simulink model "Bioloid_FK"  (R2013a)
settings: Solver=ode45  StartTime=0.0  StopTime=inf  RelTol=1e-3
undefined symbols (not defined in the file or in its folder): ToSimulink_Bioloid_FK_ST, ToSimulink_Bioloid_Signals2VRML
libraries: simulink x24, vrlib x1
settings Model: Creator=Jose Angel Rangel  LastModifiedBy=Angel

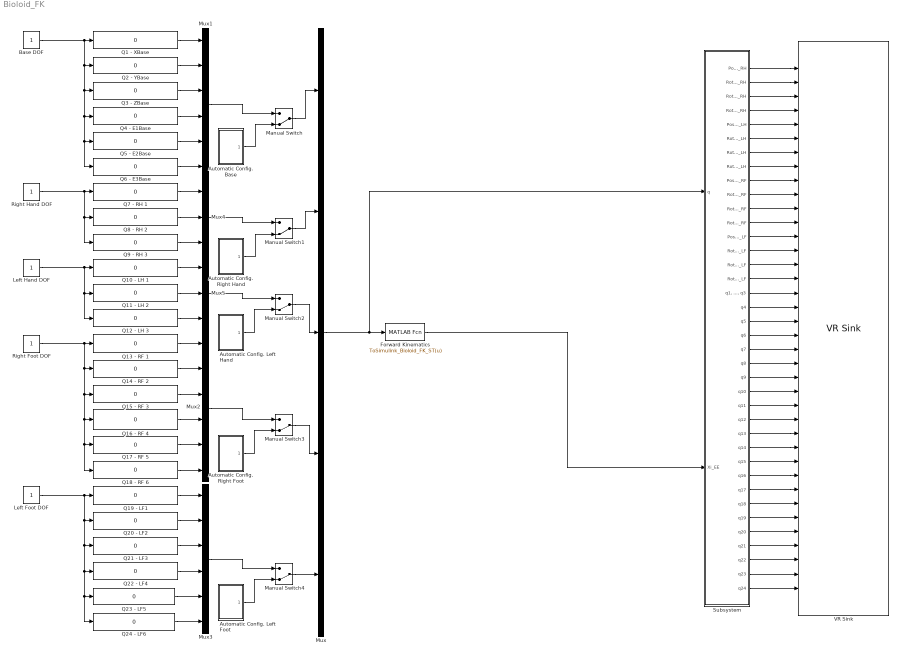
== system Bioloid_FK ==
  Automatic Config. Base : Subsystem
  Automatic Config. Left Foot : Subsystem
  Automatic Config. Left Hand : Subsystem
  Automatic Config. Right Foot : Subsystem
  Automatic Config. Right Hand : Subsystem
  Base DOF : Constant
  Forward Kinematics : MATLABFcn  MATLABFcn=ToSimulink_Bioloid_FK_ST(u)
  Left Foot DOF : Constant
  Left Hand DOF : Constant
  Manual Switch{,1..4} (5 alike) : ManualSwitch  CurrentSetting=0
  Mux : Mux  Inputs=5
  Mux1 : Mux  Inputs=6
  Mux2 : Mux  Inputs=6
  Mux3 : Mux  Inputs=6
  Mux4 : Mux  Inputs=3
  Mux5 : Mux  Inputs=3
  "Q1 - XBase " : simulink/Math Operations/Slider Gain  low=-6.28  gain=0  high=6.28
  Q10 - LH 1 : simulink/Math Operations/Slider Gain  low=-6.28  gain=0  high=6.28
  "Q11 - LH 2 " : simulink/Math Operations/Slider Gain  low=-6.28  gain=0  high=6.28
  Q12 - LH 3 : simulink/Math Operations/Slider Gain  low=-6.28  gain=0  high=6.28
  Q13 - RF 1 : simulink/Math Operations/Slider Gain  low=-6.28  gain=0  high=6.28
  Q14 - RF 2 : simulink/Math Operations/Slider Gain  low=-6.28  gain=0  high=6.28
  Q15 - RF 3 : simulink/Math Operations/Slider Gain  low=-6.28  gain=0  high=6.28
  Q16 - RF 4 : simulink/Math Operations/Slider Gain  low=-6.28  gain=0  high=6.28
  Q17 - RF 5 : simulink/Math Operations/Slider Gain  low=-6.28  gain=0  high=6.28
  Q18 - RF 6 : simulink/Math Operations/Slider Gain  low=-6.28  gain=0  high=6.28
  Q19 - LF1 : simulink/Math Operations/Slider Gain  low=-6.28  gain=0  high=6.28
  "Q2 - YBase " : simulink/Math Operations/Slider Gain  low=-6.28  gain=0  high=6.28
  Q20 - LF2 : simulink/Math Operations/Slider Gain  low=-6.28  gain=0  high=6.28
  Q21 - LF3 : simulink/Math Operations/Slider Gain  low=-6.28  gain=0  high=6.28
  Q22 - LF4 : simulink/Math Operations/Slider Gain  low=-6.28  gain=0  high=6.28
  Q23 - LF5 : simulink/Math Operations/Slider Gain  low=-6.28  gain=0  high=6.28
  Q24 - LF6 : simulink/Math Operations/Slider Gain  low=-6.28  gain=0  high=6.28
  "Q3 - ZBase " : simulink/Math Operations/Slider Gain  low=-6.28  gain=0  high=6.28
  "Q4 - E1Base " : simulink/Math Operations/Slider Gain  low=-6.28  gain=0  high=6.28
  "Q5 - E2Base " : simulink/Math Operations/Slider Gain  low=-6.28  gain=0  high=6.28
  Q6 - E3Base : simulink/Math Operations/Slider Gain  low=-6.28  gain=0  high=6.28
  Q7 - RH 1 : simulink/Math Operations/Slider Gain  low=-6.28  gain=0  high=6.28
  Q8 - RH 2 : simulink/Math Operations/Slider Gain  low=-6.28  gain=0  high=6.28
  "Q9 - RH 3 " : simulink/Math Operations/Slider Gain  low=-6.28  gain=0  high=6.28
  Right Foot DOF : Constant
  Right Hand DOF : Constant
  Subsystem : Subsystem
  VR Sink : vrlib/VR Sink  InstantiateOnLoad=on  SampleTime=0.1  ViewEnable=on  RemoteChange=off  RemoteView=off  FieldsWritten=EE_RH_Traslation.translation.3.1.1.double#EE_RH_RotX.rotation.4.1.1.double#EE_RH_RotY.rotation.4.1.1.double#EE_RH_RotZ.rotation.4.1.1.double#EE_LH_Traslation.translation.3.1.1.double#EE_LH_RotX.rotation.4.1.1.double#EE_LH_RotY.rotation.4.1.1.double#EE_LH_RotZ.rotation.4.1.1.double#EE_RF_Traslation.translation.3.1.1.double#EE_RF_RotX.rotation.4.1.1.double#EE_RF_RotY.rotation.4.1.1.double#EE_RF_RotZ.rotation.4.1.1.double#EE_LF_Traslation.translation.3.1.1.double#EE_LF_RotX.rotation.4.1.1.double#EE_LF_RotY.rotation.4.1.1.double#EE_LF_RotZ.rotation.4.1.1.double#TrunkTraslation.translation.3.1.1.double#TrunkRotX.rotation.4.1.1.double#TrunkRotY.rotation.4.1.1.double#TrunkRotZ.rotation.4.1.1.double#Right_Arm.rotation.4.1.1.double#Right_Humeros1.rotation.4.1.1.double#Right_Hand1.rotation.4.1.1.double#Left_Arm.rotation.4.1.1.double#Left_Humeros1.rotation.4.1.1.double#Left_Hand1.rotation.4.1.1.double#Right_Groin.rotation.4.1.1.double#Right_Hip1.rotation.4.1.1.double#Right_Femur1.rotation.4.1.1.double#Right_Tibia1.rotation.4.1.1.double#Right_Ankle1.rotation.4.1.1.double#Right_Foot1.rotation.4.1.1.double#Left_Groin.rotation.4.1.1.double#Left_Hip1.rotation.4.1.1.double#Left_Femur1.rotation.4.1.1.double#Left_Tibia1.rotation.4.1.1.double#Left_Ankle1.rotation.4.1.1.double#Left_Foot1.rotation.4.1.1.double  WorldFileName=Bioloid (Fisico White_Background).WRL  AutoView=on  VideoDimensions=[]  AllowVariableSize=off
  wires:
  Right Hand DOF/1 -> "Q9 - RH 3 "/1, Q8 - RH 2/1, Q7 - RH 1/1
  Mux/1 -> Subsystem/1(q), Forward Kinematics/1
  Forward Kinematics/1 -> Subsystem/2(Xi_EE)
  Base DOF/1 -> Q6 - E3Base/1, "Q5 - E2Base "/1, "Q4 - E1Base "/1, "Q3 - ZBase "/1, "Q2 - YBase "/1, "Q1 - XBase "/1
  Left Hand DOF/1 -> Q12 - LH 3/1, "Q11 - LH 2 "/1, Q10 - LH 1/1
  Right Foot DOF/1 -> Q18 - RF 6/1, Q17 - RF 5/1, Q16 - RF 4/1, Q15 - RF 3/1, Q14 - RF 2/1, Q13 - RF 1/1
  Left Foot DOF/1 -> Q19 - LF1/1, Q24 - LF6/1, Q23 - LF5/1, Q22 - LF4/1, Q21 - LF3/1, Q20 - LF2/1
  Q6 - E3Base/1 -> Mux1/6
  "Q5 - E2Base "/1 -> Mux1/5
  "Q4 - E1Base "/1 -> Mux1/4
  "Q3 - ZBase "/1 -> Mux1/3
  "Q2 - YBase "/1 -> Mux1/2
  "Q1 - XBase "/1 -> Mux1/1
  Q13 - RF 1/1 -> Mux2/1
  Q14 - RF 2/1 -> Mux2/2
  Q15 - RF 3/1 -> Mux2/3
  Q16 - RF 4/1 -> Mux2/4
  Q17 - RF 5/1 -> Mux2/5
  Q18 - RF 6/1 -> Mux2/6
  Q19 - LF1/1 -> Mux3/1
  Q20 - LF2/1 -> Mux3/2
  Q21 - LF3/1 -> Mux3/3
  Q22 - LF4/1 -> Mux3/4
  Q23 - LF5/1 -> Mux3/5
  Q24 - LF6/1 -> Mux3/6
  Q7 - RH 1/1 -> Mux4/1
  Q8 - RH 2/1 -> Mux4/2
  "Q9 - RH 3 "/1 -> Mux4/3
  "Q11 - LH 2 "/1 -> Mux5/2
  Q12 - LH 3/1 -> Mux5/3
  Q10 - LH 1/1 -> Mux5/1
  Automatic Config. Base/1(Base config) -> Manual Switch/2
  Manual Switch/1 -> Mux/1
  Mux1/1 -> Manual Switch/1
  Automatic Config. Right Hand/1(Right Hand Config.) -> Manual Switch1/2
  Manual Switch1/1 -> Mux/2
  Mux4/1 -> Manual Switch1/1
  Automatic Config. Left Hand/1(Left Hand Config.) -> Manual Switch2/2
  Manual Switch2/1 -> Mux/3
  Mux5/1 -> Manual Switch2/1
  Automatic Config. Right Foot/1(Right Foot Config) -> Manual Switch3/2
  Manual Switch3/1 -> Mux/4
  Mux2/1 -> Manual Switch3/1
  Automatic Config. Left Foot/1(Base config) -> Manual Switch4/2
  Manual Switch4/1 -> Mux/5
  Mux3/1 -> Manual Switch4/1
  Subsystem/1(Pos_EE_RH) -> VR Sink/1
  Subsystem/2(RotX_EE_RH) -> VR Sink/2
  Subsystem/3(RotY_EE_RH) -> VR Sink/3
  Subsystem/4(RotZ_EE_RH) -> VR Sink/4
  Subsystem/5(Pos_EE_LH) -> VR Sink/5
  Subsystem/6(RotX_EE_LH) -> VR Sink/6
  Subsystem/7(RotY_EE_LH) -> VR Sink/7
  Subsystem/8(RotZ_EE_LH) -> VR Sink/8
  Subsystem/9(Pos_EE_RF) -> VR Sink/9
  Subsystem/10(RotX_EE_RF) -> VR Sink/10
  Subsystem/11(RotY_EE_RF) -> VR Sink/11
  Subsystem/12(RotZ_EE_RF) -> VR Sink/12
  Subsystem/13(Pos_EE_LF) -> VR Sink/13
  Subsystem/14(RotX_EE_LF) -> VR Sink/14
  Subsystem/15(RotY_EE_LF) -> VR Sink/15
  Subsystem/16(RotZ_EE_LF) -> VR Sink/16
  Subsystem/17("q1, q2, q3") -> VR Sink/17
  Subsystem/18(q4) -> VR Sink/18
  Subsystem/19("q5 ") -> VR Sink/19
  Subsystem/20(q6) -> VR Sink/20
  Subsystem/21(q7) -> VR Sink/21
  Subsystem/22(q8) -> VR Sink/22
  Subsystem/23(q9) -> VR Sink/23
  Subsystem/24(q10) -> VR Sink/24
  Subsystem/25(q11) -> VR Sink/25
  Subsystem/26(q12) -> VR Sink/26
  Subsystem/27(q13) -> VR Sink/27
  Subsystem/28(q14) -> VR Sink/28
  Subsystem/29(q15) -> VR Sink/29
  Subsystem/30(q16) -> VR Sink/30
  Subsystem/31(q17) -> VR Sink/31
  Subsystem/32(q18) -> VR Sink/32
  Subsystem/33(q19) -> VR Sink/33
  Subsystem/34(q20) -> VR Sink/34
  Subsystem/35(q21) -> VR Sink/35
  Subsystem/36(q22) -> VR Sink/36
  Subsystem/37(q23) -> VR Sink/37
  Subsystem/38(q24) -> VR Sink/38

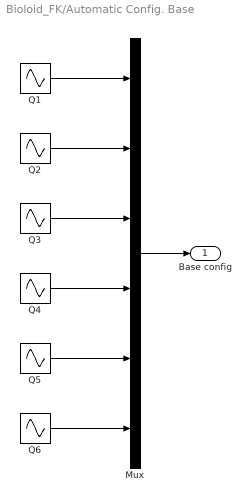
== system Bioloid_FK/Automatic Config. Base ==
  Mux : Mux  Inputs=6
  Q1 : Sin  Amplitude=3.14  Frequency=.1  SampleTime=0
  Q2 : Sin  Amplitude=3.14  Frequency=.4  SampleTime=0
  Q3 : Sin  Amplitude=3.14  Frequency=.8  SampleTime=0
  Q4 : Sin  Amplitude=3.14  Frequency=.1  SampleTime=0
  Q5 : Sin  Amplitude=3.14  Frequency=.2  SampleTime=0
  Q6 : Sin  Amplitude=3.14  Frequency=.6  SampleTime=0
  Base config : Outport
  wires:
  Mux/1 -> Base config/1
  Q5/1 -> Mux/5
  Q6/1 -> Mux/6
  Q3/1 -> Mux/3
  Q1/1 -> Mux/1
  Q2/1 -> Mux/2
  Q4/1 -> Mux/4

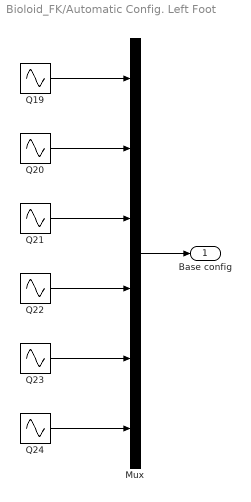
== system Bioloid_FK/Automatic Config. Left Foot ==
  Mux : Mux  Inputs=6
  Q19 : Sin  Amplitude=6.28  SampleTime=0
  Q20 : Sin  Amplitude=6.28  Frequency=.1  SampleTime=0
  Q21 : Sin  Amplitude=6.28  Frequency=.5  SampleTime=0
  Q22 : Sin  Amplitude=6.28  Frequency=.5  SampleTime=0
  Q23 : Sin  Amplitude=6.28  SampleTime=0
  Q24 : Sin  Amplitude=6.28  Frequency=.1  SampleTime=0
  Base config : Outport
  wires:
  Mux/1 -> Base config/1
  Q23/1 -> Mux/5
  Q24/1 -> Mux/6
  Q21/1 -> Mux/3
  Q19/1 -> Mux/1
  Q20/1 -> Mux/2
  Q22/1 -> Mux/4

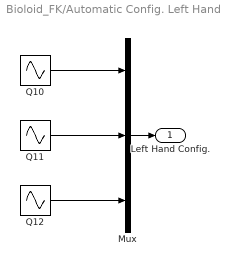
== system Bioloid_FK/Automatic Config. Left Hand ==
  Mux : Mux  Inputs=3
  Q10 : Sin  Amplitude=6.28  SampleTime=0
  Q11 : Sin  Amplitude=6.28  Frequency=.5  SampleTime=0
  Q12 : Sin  Amplitude=6.28  Frequency=.1  SampleTime=0
  Left Hand Config. : Outport
  wires:
  Mux/1 -> Left Hand Config./1
  Q12/1 -> Mux/3
  Q11/1 -> Mux/2
  Q10/1 -> Mux/1

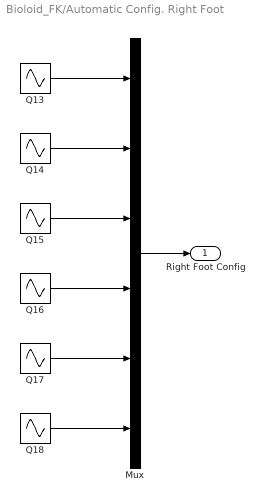
== system Bioloid_FK/Automatic Config. Right Foot ==
  Mux : Mux  Inputs=6
  Q13 : Sin  Amplitude=6.28  Frequency=.1  SampleTime=0
  Q14 : Sin  Amplitude=6.28  Frequency=.5  SampleTime=0
  Q15 : Sin  Amplitude=6.28  SampleTime=0
  Q16 : Sin  Amplitude=6.28  Frequency=.1  SampleTime=0
  Q17 : Sin  Amplitude=6.28  Frequency=.5  SampleTime=0
  Q18 : Sin  Amplitude=6.28  SampleTime=0
  Right Foot Config : Outport
  wires:
  Mux/1 -> Right Foot Config/1
  Q17/1 -> Mux/5
  Q18/1 -> Mux/6
  Q15/1 -> Mux/3
  Q13/1 -> Mux/1
  Q14/1 -> Mux/2
  Q16/1 -> Mux/4

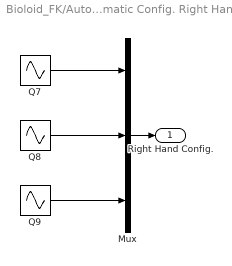
== system Bioloid_FK/Automatic Config. Right Hand ==
  Mux : Mux  Inputs=3
  Q7 : Sin  Amplitude=6.28  Frequency=.1  SampleTime=0
  Q8 : Sin  Amplitude=6.28  Frequency=.5  SampleTime=0
  Q9 : Sin  Amplitude=6.28  SampleTime=0
  Right Hand Config. : Outport
  wires:
  Mux/1 -> Right Hand Config./1
  Q9/1 -> Mux/3
  Q8/1 -> Mux/2
  Q7/1 -> Mux/1

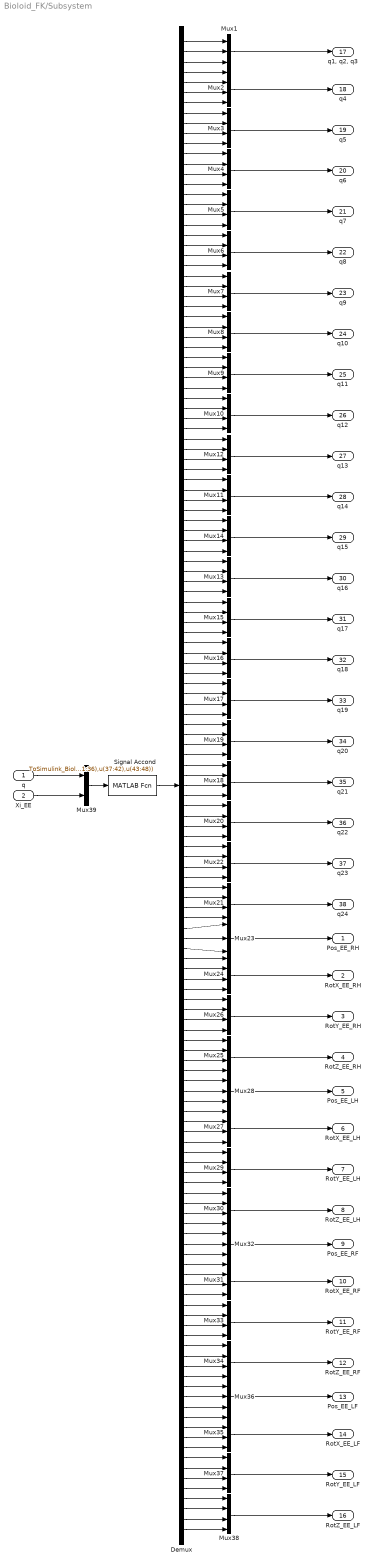
== system Bioloid_FK/Subsystem ==
  q : Inport
  Xi_EE : Inport  Port=2
  Demux : Demux  Outputs=147
  Mux{1,23,28,32,36} (5 alike) : Mux  Inputs=3
  Mux{2..22,24..27,29..31,33..35,37..38} (33 alike) : Mux
  Mux39 : Mux  Inputs=2
  Signal Accond : MATLABFcn  MATLABFcn=ToSimulink_Bioloid_Signals2VRML(u(1:24),u(25:30),u(31:36),u(37:42),u(43:48))
  Pos_EE_RH : Outport
  RotX_EE_RH : Outport  Port=2
  RotY_EE_RH : Outport  Port=3
  RotZ_EE_RH : Outport  Port=4
  Pos_EE_LH : Outport  Port=5
  RotX_EE_LH : Outport  Port=6
  RotY_EE_LH : Outport  Port=7
  RotZ_EE_LH : Outport  Port=8
  Pos_EE_RF : Outport  Port=9
  RotX_EE_RF : Outport  Port=10
  RotY_EE_RF : Outport  Port=11
  RotZ_EE_RF : Outport  Port=12
  Pos_EE_LF : Outport  Port=13
  RotX_EE_LF : Outport  Port=14
  RotY_EE_LF : Outport  Port=15
  RotZ_EE_LF : Outport  Port=16
  "q1, q2, q3" : Outport  Port=17
  q4 : Outport  Port=18
  "q5 " : Outport  Port=19
  q6 : Outport  Port=20
  q7 : Outport  Port=21
  q8 : Outport  Port=22
  q9 : Outport  Port=23
  q10 : Outport  Port=24
  q11 : Outport  Port=25
  q12 : Outport  Port=26
  q13 : Outport  Port=27
  q14 : Outport  Port=28
  q15 : Outport  Port=29
  q16 : Outport  Port=30
  q17 : Outport  Port=31
  q18 : Outport  Port=32
  q19 : Outport  Port=33
  q20 : Outport  Port=34
  q21 : Outport  Port=35
  q22 : Outport  Port=36
  q23 : Outport  Port=37
  q24 : Outport  Port=38
  wires:
  Demux/7 -> Mux2/4
  Mux11/1 -> q14/1
  Demux/4 -> Mux2/1
  Mux38/1 -> RotZ_EE_LF/1
  Mux10/1 -> q12/1
  Demux/1 -> Mux1/1
  Demux/3 -> Mux1/3
  Mux18/1 -> q21/1
  Demux/6 -> Mux2/3
  Mux1/1 -> "q1, q2, q3"/1
  Mux15/1 -> q17/1
  Mux8/1 -> q10/1
  Demux/5 -> Mux2/2
  Demux/2 -> Mux1/2
  Demux/8 -> Mux3/1
  Mux28/1 -> Pos_EE_LH/1
  Mux16/1 -> q18/1
  Mux3/1 -> "q5 "/1
  Mux7/1 -> q9/1
  Mux14/1 -> q15/1
  Mux9/1 -> q11/1
  Mux22/1 -> q23/1
  Mux2/1 -> q4/1
  Mux4/1 -> q6/1
  Mux5/1 -> q7/1
  Mux30/1 -> RotZ_EE_LH/1
  Mux13/1 -> q16/1
  Mux12/1 -> q13/1
  Mux24/1 -> RotX_EE_RH/1
  Mux20/1 -> q22/1
  Mux19/1 -> q20/1
  Mux6/1 -> q8/1
  Mux25/1 -> RotZ_EE_RH/1
  Mux17/1 -> q19/1
  Mux26/1 -> RotY_EE_RH/1
  Mux21/1 -> q24/1
  Mux23/1 -> Pos_EE_RH/1
  Mux36/1 -> Pos_EE_LF/1
  Mux32/1 -> Pos_EE_RF/1
  Mux31/1 -> RotX_EE_RF/1
  Mux33/1 -> RotY_EE_RF/1
  Mux35/1 -> RotX_EE_LF/1
  Mux34/1 -> RotZ_EE_RF/1
  Mux37/1 -> RotY_EE_LF/1
  Mux27/1 -> RotX_EE_LH/1
  Mux29/1 -> RotY_EE_LH/1
  Demux/10 -> Mux3/3
  Demux/9 -> Mux3/2
  Demux/11 -> Mux3/4
  Demux/12 -> Mux4/1
  Demux/15 -> Mux4/4
  Demux/13 -> Mux4/2
  Demux/14 -> Mux4/3
  Signal Accond/1 -> Demux/1
  q/1 -> Mux39/1
  Xi_EE/1 -> Mux39/2
  Mux39/1 -> Signal Accond/1
  Demux/55 -> Mux13/4
  Demux/50 -> Mux14/3
  Demux/70 -> Mux19/3
  Demux/45 -> Mux11/2
  Demux/37 -> Mux10/2
  Demux/28 -> Mux8/1
  Demux/35 -> Mux9/4
  Demux/40 -> Mux12/1
  Demux/27 -> Mux7/4
  Demux/41 -> Mux12/2
  Demux/46 -> Mux11/3
  Demux/69 -> Mux19/2
  Demux/58 -> Mux15/3
  Demux/33 -> Mux9/2
  Demux/20 -> Mux6/1
  Demux/66 -> Mux17/3
  Demux/36 -> Mux10/1
  Demux/26 -> Mux7/3
  Demux/59 -> Mux15/4
  Demux/49 -> Mux14/2
  Demux/47 -> Mux11/4
  Demux/60 -> Mux16/1
  Demux/38 -> Mux10/3
  Demux/63 -> Mux16/4
  Demux/54 -> Mux13/3
  Demux/18 -> Mux5/3
  Demux/34 -> Mux9/3
  Demux/44 -> Mux11/1
  Demux/29 -> Mux8/2
  Demux/51 -> Mux14/4
  Demux/31 -> Mux8/4
  Demux/30 -> Mux8/3
  Demux/64 -> Mux17/1
  Demux/16 -> Mux5/1
  Demux/53 -> Mux13/2
  Demux/52 -> Mux13/1
  Demux/17 -> Mux5/2
  Demux/22 -> Mux6/3
  Demux/48 -> Mux14/1
  Demux/43 -> Mux12/4
  Demux/25 -> Mux7/2
  Demux/24 -> Mux7/1
  Demux/32 -> Mux9/1
  Demux/56 -> Mux15/1
  Demux/39 -> Mux10/4
  Demux/23 -> Mux6/4
  Demux/21 -> Mux6/2
  Demux/61 -> Mux16/2
  Demux/19 -> Mux5/4
  Demux/42 -> Mux12/3
  Demux/67 -> Mux17/4
  Demux/65 -> Mux17/2
  Demux/57 -> Mux15/2
  Demux/62 -> Mux16/3
  Demux/68 -> Mux19/1
  Demux/113 -> Mux29/4
  Demux/86 -> Mux21/3
  Demux/143 -> Mux37/4
  Demux/107 -> Mux27/2
  Demux/112 -> Mux29/3
  Demux/131 -> Mux34/3
  Demux/133 -> Mux36/1
  Demux/126 -> Mux33/2
  Demux/139 -> Mux35/4
  Demux/83 -> Mux22/4
  Demux/72 -> Mux18/1
  Demux/134 -> Mux36/2
  Demux/137 -> Mux35/2
  Demux/115 -> Mux30/2
  Demux/132 -> Mux34/4
  Demux/125 -> Mux33/1
  Demux/71 -> Mux19/4
  Demux/89 -> Mux23/2
  Demux/128 -> Mux33/4
  Demux/144 -> Mux38/1
  Demux/77 -> Mux20/2
  Demux/118 -> Mux32/1
  Demux/103 -> Mux28/1
  Demux/101 -> Mux25/3
  Demux/100 -> Mux25/2
  Demux/78 -> Mux20/3
  Demux/98 -> Mux26/4
  Demux/142 -> Mux37/3
  Demux/102 -> Mux25/4
  Demux/138 -> Mux35/3
  Demux/123 -> Mux31/3
  Demux/96 -> Mux26/2
  Demux/145 -> Mux38/2
  Demux/99 -> Mux25/1
  Demux/122 -> Mux31/2
  Demux/84 -> Mux21/1
  Demux/116 -> Mux30/3
  Demux/114 -> Mux30/1
  Demux/88 -> Mux23/1
  Demux/108 -> Mux27/3
  Demux/121 -> Mux31/1
  Demux/120 -> Mux32/3
  Demux/76 -> Mux20/1
  Demux/90 -> Mux23/3
  Demux/147 -> Mux38/4
  Demux/111 -> Mux29/2
  Demux/85 -> Mux21/2
  Demux/79 -> Mux20/4
  Demux/93 -> Mux24/3
  Demux/74 -> Mux18/3
  Demux/109 -> Mux27/4
  Demux/136 -> Mux35/1
  Demux/87 -> Mux21/4
  Demux/127 -> Mux33/3
  Demux/82 -> Mux22/3
  Demux/146 -> Mux38/3
  Demux/80 -> Mux22/1
  Demux/81 -> Mux22/2
  Demux/75 -> Mux18/4
  Demux/97 -> Mux26/3
  Demux/91 -> Mux24/1
  Demux/95 -> Mux26/1
  Demux/124 -> Mux31/4
  Demux/105 -> Mux28/3
  Demux/73 -> Mux18/2
  Demux/104 -> Mux28/2
  Demux/94 -> Mux24/4
  Demux/92 -> Mux24/2
  Demux/135 -> Mux36/3
  Demux/110 -> Mux29/1
  Demux/130 -> Mux34/2
  Demux/140 -> Mux37/1
  Demux/141 -> Mux37/2
  Demux/117 -> Mux30/4
  Demux/129 -> Mux34/1
  Demux/119 -> Mux32/2
  Demux/106 -> Mux27/1
